simulink model "floating_2_bodies_acc"  (Simulink 6.3)
settings: Solver=ode1  StartTime=0.0  StopTime=inf  FixedStep=0.01  RelTol=1e-6  AbsTol=1e-6
PreLoadFcn:
  | Body_Shv_Double_0661
InitFcn:
  | mech_slider_open_ShV(gcs);
undefined symbols (not defined in the file): Body_01_Inertia, Body_01_Mass, Body_Rt_Inertia, Body_Rt_Mass, deg, Range_of_Ang_degr, s
libraries: mblibv1 x23, simulink x11
settings Model: LastModifiedBy=Alex
settings SimMechanicsCC: VisOnUpdateDiagram=on  VisDuringSimulation=on

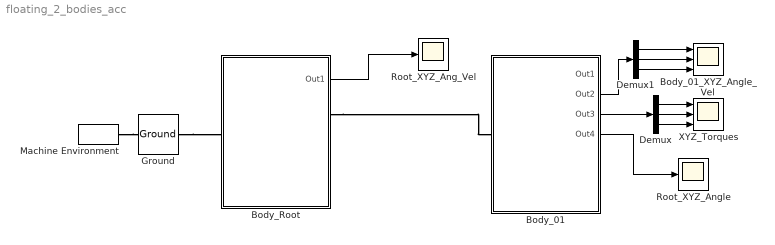
== system floating_2_bodies_acc ==
  Body_01 : Subsystem
  Body_01_XYZ_Angle_Vel : Scope  NumInputPorts=3
      settings: TimeRange=30  YMin=-8e-005~-1~-1  YMax=2e-005~1~1
  Body_Root : Subsystem
  Demux : Demux  Outputs=3
  Demux1 : Demux  Outputs=3
  Ground : mblibv1/Bodies/Ground  LeftPortType=env  RightPortType=workingframe  PhysicalDomain=Mechanical  DialogClass=GroundBlock  CoordPosition=[0 0 0]  CoordPositionUnits=m  StateVectorMgrId=-1  MachineId=[6 1]  ShowEnvPort=on
  Machine Environment : mblibv1/Bodies/Machine Environment  Tag=Factory ground  DialogController=MECH.DialogSource  PortType=env  PhysicalDomain=Mechanical  DialogTemplateClass=MECH.MachineEnvironment  SyncWhenCopied=off  Gravity=[0 0 0]  GravityUnits=m/s^2  GravityAsSignal=off  Dimensionality=Auto-detect  AnalysisType=Forward dynamics  LinearAssemblyTolerance=1e-3  LinearAssemblyToleranceUnits=m  AngularAssemblyTolerance=1e-3  AngularAssemblyToleranceUnits=rad  ConstraintSolverType=Stabilizing  ConstraintRelTolerance=1e-4  ConstraintAbsTolerance=1e-4  UseRobustSingularityHandling=off  StatePerturbationType=Fixed  PerturbationSize=1e-5  VisualizeMachine=on
  Root_XYZ_Ang_Vel : Scope
      settings: TimeRange=60  YMin=-600  YMax=700
  Root_XYZ_Angle : Scope
      settings: TimeRange=10  YMin=-90  YMax=10  SaveName=ScopeData4
  XYZ_Torques : Scope  NumInputPorts=3
      settings: TimeRange=30  YMin=1.01794~-1~-1  YMax=1.01797~1~1  SaveName=ScopeData3
  wires:
  Body_01/3(Out3) -> Demux/1
  Demux/1 -> XYZ_Torques/1
  Demux/2 -> XYZ_Torques/2
  Demux/3 -> XYZ_Torques/3
  Body_01/2(Out2) -> Demux1/1
  Demux1/1 -> Body_01_XYZ_Angle_Vel/1
  Demux1/2 -> Body_01_XYZ_Angle_Vel/2
  Demux1/3 -> Body_01_XYZ_Angle_Vel/3
  Body_Root/1(Out1) -> Root_XYZ_Ang_Vel/1
  Body_01/4(Out4) -> Root_XYZ_Angle/1
  connections:
  Machine Environment/RConn1 -- Ground/LConn1
  Ground/RConn1 -- Body_Root/LConn1
  Body_Root/RConn1 -- Body_01/LConn1

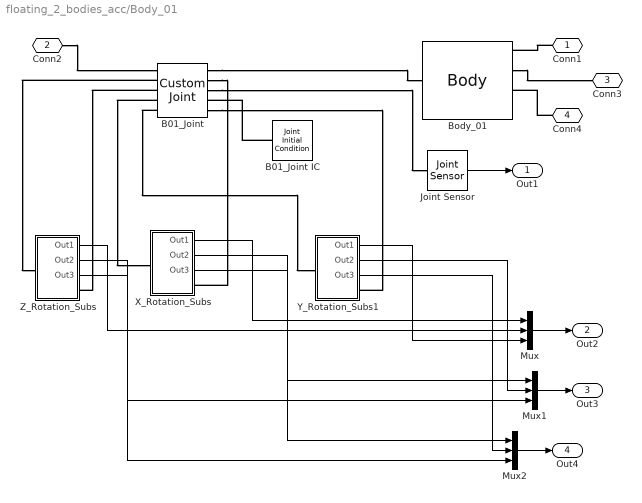
== system floating_2_bodies_acc/Body_01 ==
  B01_Joint : mblibv1/Joints/Custom Joint  PhysicalDomain=mechanical  SubClassName=custom_joint  LeftPortType=blob  RightPortType=blob  LConnTagsString=__newl0|SA1|SA2|SA3|SA4  RConnTagsString=__newr0|SA1|SA2|SA3|SA4  NumSAPorts=8  CutJoint=off  MarkAsCut=off  Primitives=revolute_revolute_revolute  PrimitiveProps=R3$WORLD$[0 0 1]$revolute#R1$WORLD$[1 0 0]$revolute#R2$WORLD$[0 1 0]$revolute  DialogClass=JointBlock
  B01_Joint IC : mblibv1/Sensors &  Actuators/Joint Initial Condition  Orientation=left  PhysicalDomain=mechanical  DialogClass=InitialConditionBlock  InitialConditions=P1$false$0$m$rad$0$m/s$rad/s#P2$false$0$m$rad$0$m/s$rad/s#P3$false$0$m$rad$0$m/s$rad/s#R1$true$X_Ang_Correction$m$deg$Body_01_IVel(1)$m/s$rad/s#R2$true$Body_01_IPos(2)$m$deg$Body_01_IVel(2)$m/s$rad/s#R3$true$Body_01_IPos(3)$m$deg$Body_01_IVel(3)$m/s$rad/s#S$false$0$m$rad$0$m/s$rad/s
  Body_01 : mblibv1/Bodies/Body  PhysicalDomain=mechanical  SubClassName=Unknown  LeftPortType=workingframe  RightPortType=workingframe  LConnTagsString=CS1  RConnTagsString=CS2|CS3|CS4|CS5  DialogClass=MechanicalBodyBlock  Mass=Body_01_Mass  MassUnits=kg  InertiaUnits=kg*m^2  Inertia=Body_01_Inertia  Shape=Cylinder  ShapeDims=[1 1]  ShapeUnits=m  ShapeUse=false  Density=1  DensityUnits=kg/m^3  DensityUse=false  CG=Left$CG$-Body_01_Size$CS1$CS1$m$[0 0 0]$Euler X-Y-Z$deg$ADJOINING$false  WorkingFrames=Left$CS1$[0 0 0]$ADJOINING$ADJOINING$m$[0 0 0]$Euler X-Y-Z$deg$WORLD$true#Right$CS2$-Body_01_Size$CG$CG$m$[0 0 0]$Euler X-Y-Z$deg$WORLD$true#Right$CS3$[-0.5*Body_01_Size(2) -Body_01_Size(2) 0]$CG$CG$m$[0 0 0]$Euler X-Y-Z$deg$WORLD$true#Right$CS4$[0.5*Body_01_Size(2) -Body_01_Size(2) 0]$CG$CG$m$[0 0 0]$Euler X-Y-Z$deg$WORLD$true#Right$CS5$[0 -Body_01_Size(2) -0.2*Body_01_Size(2)]$CG$CG$m$[0 0 0]$Euler X-Y-Z$deg$WORLD$true
  Joint Sensor : mblibv1/Sensors &  Actuators/Joint Sensor  PhysicalDomain=Mechanical  PortType=blob  Muxed=on  Pose=off  Angle=off  AngleUnits=deg  ArcVelocity=on  ArcVelocityUnits=deg/s  ArcAcceleration=off  ArcAccelerationUnits=deg/s^2  CoordPosition=on  CoordPositionUnits=m  Velocity=off  VelocityUnits=m/s  Acceleration=off  AccelerationUnits=m/s^2  Quaternion=on  QuaternionDT=off  QuaternionDDT=off  QuaternionUnits=off  OutputVector=[ 1 ]  ActiveIO=on  Width=1  DialogClass=MechanicalSensorBlock  Primitive=R3  Force=off  ForceUnits=N  Torque=off  TorqueUnits=N-m  ReferenceFrame=Absolute (INERTIAL)  ReactionSensedSide=Base  ReactionReferenceFrame=Local (Body CS)  ReactionForce=off  ReactionForceUnits=N  ReactionMoment=off  ReactionMomentUnits=N-m
  Mux : Mux  Inputs=3
  Mux1 : Mux  Inputs=3
  Mux2 : Mux  Inputs=3
  X_Rotation_Subs : Subsystem
  Y_Rotation_Subs1 : Subsystem
  Z_Rotation_Subs : Subsystem
  Conn1 : PMIOPort  Orientation=left  Port=1  Side=Right
  Conn2 : PMIOPort  Port=2  Side=Left
  Conn3 : PMIOPort  Orientation=left  Port=3  Side=Right
  Conn4 : PMIOPort  Orientation=left  Port=4  Side=Right
  Out1 : Outport
  Out2 : Outport  Port=2
  Out3 : Outport  Port=3
  Out4 : Outport  Port=4
  wires:
  Joint Sensor/1 -> Out1/1
  Z_Rotation_Subs/1(Out1) -> Mux/2
  X_Rotation_Subs/1(Out1) -> Mux/1
  Mux/1 -> Out2/1
  Y_Rotation_Subs1/1(Out1) -> Mux/3
  Mux1/1 -> Out3/1
  X_Rotation_Subs/2(Out2) -> Mux1/1
  Y_Rotation_Subs1/2(Out2) -> Mux1/2
  Z_Rotation_Subs/2(Out2) -> Mux1/3
  Mux2/1 -> Out4/1
  X_Rotation_Subs/3(Out3) -> Mux2/1
  Y_Rotation_Subs1/3(Out3) -> Mux2/2
  Z_Rotation_Subs/3(Out3) -> Mux2/3
  connections:
  B01_Joint/RConn1 -- Body_01/LConn1
  B01_Joint/RConn3 -- Joint Sensor/LConn1
  Conn1/RConn1 -- Body_01/RConn1
  Conn2/RConn1 -- B01_Joint/LConn1
  Conn4/RConn1 -- Body_01/RConn3
  B01_Joint/LConn2 -- Z_Rotation_Subs/LConn1
  B01_Joint/LConn3 -- Z_Rotation_Subs/RConn1
  B01_Joint/LConn4 -- X_Rotation_Subs/LConn1
  B01_Joint/RConn2 -- X_Rotation_Subs/RConn1
  B01_Joint IC/RConn1 -- B01_Joint/RConn4
  B01_Joint/LConn5 -- Y_Rotation_Subs1/LConn1
  B01_Joint/RConn5 -- Y_Rotation_Subs1/RConn1
  Body_01/RConn2 -- Conn3/RConn1

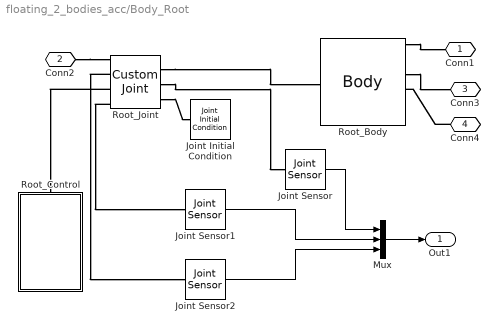
== system floating_2_bodies_acc/Body_Root ==
  Joint Initial Condition : mblibv1/Sensors &  Actuators/Joint Initial Condition  Orientation=left  PhysicalDomain=mechanical  DialogClass=InitialConditionBlock  InitialConditions=P1$true$0$m$rad$Body_Rt_IVel(1)$m/s$rad/s#P2$true$0$m$rad$Body_Rt_IVel(2)$m/s$rad/s#P3$true$0$m$rad$Body_Rt_IVel(3)$m/s$rad/s#R1$true$Body_Rt_IPos(4)$m$deg$Body_Rt_IVel(4)$m/s$rad/s#R2$true$Body_Rt_IPos(5)$m$deg$Body_Rt_IVel(5)$m/s$rad/s#R3$true$Body_Rt_IPos(6)$m$deg$Body_Rt_IVel(6)$m/s$rad/s#S$false$0$m$rad$0$m/s$rad/s
  Joint Sensor : mblibv1/Sensors &  Actuators/Joint Sensor  PhysicalDomain=Mechanical  PortType=blob  Muxed=on  Pose=off  Angle=off  AngleUnits=deg  ArcVelocity=on  ArcVelocityUnits=deg/s  ArcAcceleration=off  ArcAccelerationUnits=deg/s^2  CoordPosition=on  CoordPositionUnits=m  Velocity=off  VelocityUnits=m/s  Acceleration=off  AccelerationUnits=m/s^2  Quaternion=on  QuaternionDT=off  QuaternionDDT=off  QuaternionUnits=off  OutputVector=[ 1 ]  ActiveIO=on  Width=1  DialogClass=MechanicalSensorBlock  Primitive=R1  Force=off  ForceUnits=N  Torque=off  TorqueUnits=N-m  ReferenceFrame=Absolute (INERTIAL)  ReactionSensedSide=Base  ReactionReferenceFrame=Local (Body CS)  ReactionForce=off  ReactionForceUnits=N  ReactionMoment=off  ReactionMomentUnits=N-m
  Joint Sensor1 : mblibv1/Sensors &  Actuators/Joint Sensor  PhysicalDomain=Mechanical  PortType=blob  Muxed=on  Pose=off  Angle=off  AngleUnits=deg  ArcVelocity=on  ArcVelocityUnits=deg/s  ArcAcceleration=off  ArcAccelerationUnits=deg/s^2  CoordPosition=on  CoordPositionUnits=m  Velocity=off  VelocityUnits=m/s  Acceleration=off  AccelerationUnits=m/s^2  Quaternion=on  QuaternionDT=off  QuaternionDDT=off  QuaternionUnits=off  OutputVector=[ 1 ]  ActiveIO=on  Width=1  DialogClass=MechanicalSensorBlock  Primitive=R2  Force=off  ForceUnits=N  Torque=off  TorqueUnits=N-m  ReferenceFrame=Absolute (INERTIAL)  ReactionSensedSide=Base  ReactionReferenceFrame=Local (Body CS)  ReactionForce=off  ReactionForceUnits=N  ReactionMoment=off  ReactionMomentUnits=N-m
  Joint Sensor2 : mblibv1/Sensors &  Actuators/Joint Sensor  PhysicalDomain=Mechanical  PortType=blob  Muxed=on  Pose=off  Angle=off  AngleUnits=deg  ArcVelocity=on  ArcVelocityUnits=deg/s  ArcAcceleration=off  ArcAccelerationUnits=deg/s^2  CoordPosition=on  CoordPositionUnits=m  Velocity=off  VelocityUnits=m/s  Acceleration=off  AccelerationUnits=m/s^2  Quaternion=on  QuaternionDT=off  QuaternionDDT=off  QuaternionUnits=off  OutputVector=[ 1 ]  ActiveIO=on  Width=1  DialogClass=MechanicalSensorBlock  Primitive=R3  Force=off  ForceUnits=N  Torque=off  TorqueUnits=N-m  ReferenceFrame=Absolute (INERTIAL)  ReactionSensedSide=Base  ReactionReferenceFrame=Local (Body CS)  ReactionForce=off  ReactionForceUnits=N  ReactionMoment=off  ReactionMomentUnits=N-m
  Mux : Mux  Inputs=3
  Root_Body : mblibv1/Bodies/Body  PhysicalDomain=mechanical  SubClassName=Unknown  LeftPortType=workingframe  RightPortType=workingframe  LConnTagsString=CG  RConnTagsString=CS1|CS2|CS3|CS4|CS5|CS6  DialogClass=MechanicalBodyBlock  Mass=Body_Rt_Mass  MassUnits=kg  InertiaUnits=kg*m^2  Inertia=Body_Rt_Inertia  Shape=Cylinder  ShapeDims=[1 1]  ShapeUnits=m  ShapeUse=false  Density=1  DensityUnits=kg/m^3  DensityUse=false  CG=Left$CG$Body_Rt_IPos(1:3)$WORLD$WORLD$m$[0 0 0]$Euler X-Y-Z$deg$WORLD$true  WorkingFrames=Right$CS1$Body_Rt_Size$CG$CG$m$[0 0 0]$Euler X-Y-Z$deg$WORLD$true#Right$CS2$[0 -Body_Rt_Size(2) 0]$CG$CG$m$[0 0 0]$Euler X-Y-Z$deg$WORLD$true#Right$CS3$[-0.4*Body_Rt_Size(2) Body_Rt_Size(2) 0]$CG$CG$m$[0 0 0]$Euler X-Y-Z$deg$WORLD$true#Right$CS4$[0.4*Body_Rt_Size(2) Body_Rt_Size(2) 0]$CG$CG$m$[0 0 0]$Euler X-Y-Z$deg$WORLD$true#Right$CS5$[0 Body_Rt_Size(2) -0.2*Body_Rt_Size(2)]$CG$CG$m$[0 0 0]$Euler X-Y-Z$deg$WORLD$true#Right$CS6$-CM_loc_Rel_Rt$CG$CG$m$[0 0 0]$Euler X-Y-Z$deg$WORLD$true
  Root_Control : Subsystem  Orientation=down
  Root_Joint : mblibv1/Joints/Custom Joint  PhysicalDomain=mechanical  SubClassName=custom_joint  LeftPortType=blob  RightPortType=blob  LConnTagsString=__newl0|SA1|SA2|SA3  RConnTagsString=__newr0|SA1|SA2  NumSAPorts=5  CutJoint=off  MarkAsCut=off  Primitives=prismatic_prismatic_prismatic_revolute_revolute_revolute  PrimitiveProps=P1$WORLD$[1 0 0]$prismatic#P2$WORLD$[0 1 0]$prismatic#P3$WORLD$[0 0 1]$prismatic#R1$WORLD$[1 0 0]$revolute#R2$WORLD$[0 1 0]$revolute#R3$WORLD$[0 0 1]$revolute  DialogClass=JointBlock
  Conn1 : PMIOPort  Orientation=left  Port=1  Side=Right
  Conn2 : PMIOPort  Port=2  Side=Left
  Conn3 : PMIOPort  Orientation=left  Port=3  Side=Right
  Conn4 : PMIOPort  Orientation=left  Port=4  Side=Right
  Out1 : Outport
  wires:
  Mux/1 -> Out1/1
  Joint Sensor/1 -> Mux/1
  Joint Sensor1/1 -> Mux/2
  Joint Sensor2/1 -> Mux/3
  connections:
  Root_Joint/RConn2 -- Joint Sensor/LConn1
  Conn2/RConn1 -- Root_Joint/LConn1
  Conn4/RConn1 -- Root_Body/RConn4
  Root_Body/RConn3 -- Conn3/RConn1
  Root_Joint/RConn1 -- Root_Body/LConn1
  Root_Body/RConn1 -- Conn1/RConn1
  Root_Joint/RConn3 -- Joint Initial Condition/RConn1
  Root_Joint/LConn3 -- Root_Control/LConn1
  Root_Joint/LConn2 -- Joint Sensor2/LConn1
  Root_Joint/LConn4 -- Joint Sensor1/LConn1

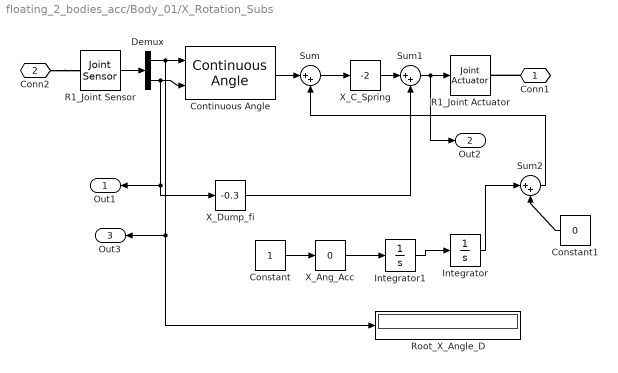
== system floating_2_bodies_acc/Body_01/X_Rotation_Subs ==
  Constant : Constant
  Constant1 : Constant  Orientation=left  Value=0
  Continuous Angle : mblibv1/Utilities/Continuous Angle  Tag=Factory continuousAngle  rad=deg  rads=deg/s
  Demux : Demux  Outputs=2
  Integrator : Integrator  LimitOutput=on  UpperSaturationLimit=Range_of_Ang_degr(2,1)  LowerSaturationLimit=Range_of_Ang_degr(1,1)
  Integrator1 : Integrator  LimitOutput=on  UpperSaturationLimit=200  LowerSaturationLimit=-200
  R1_Joint Actuator : mblibv1/Sensors &  Actuators/Joint Actuator  PhysicalDomain=Mechanical  PortType=blob  ActuationStyle=Force  AngleUnits=deg  ArcVelocityUnits=deg/s  ArcAccelerationUnits=deg/s^2  CoordPositionUnits=m  VelocityUnits=m/s  AccelerationUnits=m/s^2  ForceUnits=N  TorqueUnits=N-m  ActiveIO=on  Width=1  DialogClass=MechanicalActuatorBlock  Primitive=R1  ReferenceFrame=Absolute (INERTIAL)
  R1_Joint Sensor : mblibv1/Sensors &  Actuators/Joint Sensor  PhysicalDomain=Mechanical  PortType=blob  Muxed=on  Pose=off  Angle=on  AngleUnits=deg  ArcVelocity=on  ArcVelocityUnits=deg/s  ArcAcceleration=off  ArcAccelerationUnits=deg/s^2  CoordPosition=on  CoordPositionUnits=m  Velocity=off  VelocityUnits=m/s  Acceleration=off  AccelerationUnits=m/s^2  Quaternion=on  QuaternionDT=off  QuaternionDDT=off  QuaternionUnits=off  OutputVector=[ 1 1 ]  ActiveIO=on  Width=2  DialogClass=MechanicalSensorBlock  Primitive=R1  Force=off  ForceUnits=N  Torque=off  TorqueUnits=N-m  ReferenceFrame=Absolute (INERTIAL)  ReactionSensedSide=Base  ReactionReferenceFrame=Local (Body CS)  ReactionForce=off  ReactionForceUnits=N  ReactionMoment=off  ReactionMomentUnits=N-m
  Root_X_Angle_D : Display
  Sum : Sum  Inputs=|++
  Sum1 : Sum  Inputs=|++
  Sum2 : Sum  Inputs=|++
  X_Ang_Acc : simulink/Math Operations/Slider Gain  Tag=Start_Open  low=-1000  gain=0  high=1000
  X_C_Spring : simulink/Math Operations/Slider Gain  low=-2  gain=-2  high=0
  X_Dump_fi : simulink/Math Operations/Slider Gain  low=-0.3  gain=-0.3  high=0
  Conn1 : PMIOPort  Orientation=left  Port=1  Side=Right
  Conn2 : PMIOPort  Port=2  Side=Left
  Out1 : Outport  Orientation=left
  Out2 : Outport  Port=2
  Out3 : Outport  Orientation=left  Port=3
  wires:
  R1_Joint Sensor/1 -> Demux/1
  X_Dump_fi/1 -> Sum1/2
  Constant/1 -> X_Ang_Acc/1
  Sum/1 -> X_C_Spring/1
  X_C_Spring/1 -> Sum1/1
  Demux/1 -> Continuous Angle/1, Root_X_Angle_D/1, Out3/1
  Continuous Angle/1 -> Sum/1
  Demux/2 -> Continuous Angle/2, X_Dump_fi/1, Out1/1
  Sum1/1 -> R1_Joint Actuator/1, Out2/1
  Constant1/1 -> Sum2/2
  Integrator/1 -> Sum2/1
  Sum2/1 -> Sum/2
  Integrator1/1 -> Integrator/1
  X_Ang_Acc/1 -> Integrator1/1
  connections:
  Conn1/RConn1 -- R1_Joint Actuator/RConn1
  Conn2/RConn1 -- R1_Joint Sensor/LConn1

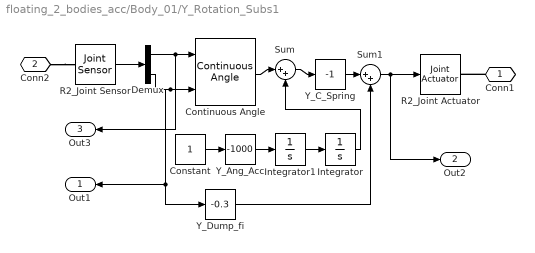
== system floating_2_bodies_acc/Body_01/Y_Rotation_Subs1 ==
  Constant : Constant
  Continuous Angle : mblibv1/Utilities/Continuous Angle  Tag=Factory continuousAngle  rad=deg  rads=deg/s
  Demux : Demux  Outputs=2
  Integrator : Integrator  LimitOutput=on  UpperSaturationLimit=Range_of_Ang_degr(2,2)  LowerSaturationLimit=Range_of_Ang_degr(1,2)
  Integrator1 : Integrator  LimitOutput=on  UpperSaturationLimit=200  LowerSaturationLimit=-200
  R2_Joint Actuator : mblibv1/Sensors &  Actuators/Joint Actuator  PhysicalDomain=Mechanical  PortType=blob  ActuationStyle=Force  AngleUnits=deg  ArcVelocityUnits=deg/s  ArcAccelerationUnits=deg/s^2  CoordPositionUnits=m  VelocityUnits=m/s  AccelerationUnits=m/s^2  ForceUnits=N  TorqueUnits=N-m  ActiveIO=on  Width=1  DialogClass=MechanicalActuatorBlock  Primitive=R2  ReferenceFrame=Absolute (INERTIAL)
  R2_Joint Sensor : mblibv1/Sensors &  Actuators/Joint Sensor  PhysicalDomain=Mechanical  PortType=blob  Muxed=on  Pose=off  Angle=on  AngleUnits=deg  ArcVelocity=on  ArcVelocityUnits=deg/s  ArcAcceleration=off  ArcAccelerationUnits=deg/s^2  CoordPosition=on  CoordPositionUnits=m  Velocity=off  VelocityUnits=m/s  Acceleration=off  AccelerationUnits=m/s^2  Quaternion=on  QuaternionDT=off  QuaternionDDT=off  QuaternionUnits=off  OutputVector=[ 1 1 ]  ActiveIO=on  Width=2  DialogClass=MechanicalSensorBlock  Primitive=R2  Force=off  ForceUnits=N  Torque=off  TorqueUnits=N-m  ReferenceFrame=Absolute (INERTIAL)  ReactionSensedSide=Base  ReactionReferenceFrame=Local (Body CS)  ReactionForce=off  ReactionForceUnits=N  ReactionMoment=off  ReactionMomentUnits=N-m
  Sum : Sum  Inputs=|++
  Sum1 : Sum  Inputs=|++
  Y_Ang_Acc : simulink/Math Operations/Slider Gain  Tag=Start_Open  low=-1000  gain=-1000  high=1000
  Y_C_Spring : simulink/Math Operations/Slider Gain  low=-1  gain=-1  high=0
  Y_Dump_fi : simulink/Math Operations/Slider Gain  low=-0.3  gain=-0.3  high=0
  Conn1 : PMIOPort  Orientation=left  Port=1  Side=Right
  Conn2 : PMIOPort  Port=2  Side=Left
  Out1 : Outport  Orientation=left
  Out2 : Outport  Port=2
  Out3 : Outport  Orientation=left  Port=3
  wires:
  R2_Joint Sensor/1 -> Demux/1
  Demux/2 -> Continuous Angle/2, Y_Dump_fi/1, Out1/1
  Y_Dump_fi/1 -> Sum1/2
  Sum1/1 -> R2_Joint Actuator/1, Out2/1
  Constant/1 -> Y_Ang_Acc/1
  Sum/1 -> Y_C_Spring/1
  Y_C_Spring/1 -> Sum1/1
  Demux/1 -> Continuous Angle/1, Out3/1
  Continuous Angle/1 -> Sum/1
  Integrator/1 -> Sum/2
  Y_Ang_Acc/1 -> Integrator1/1
  Integrator1/1 -> Integrator/1
  connections:
  Conn1/RConn1 -- R2_Joint Actuator/RConn1
  Conn2/RConn1 -- R2_Joint Sensor/LConn1

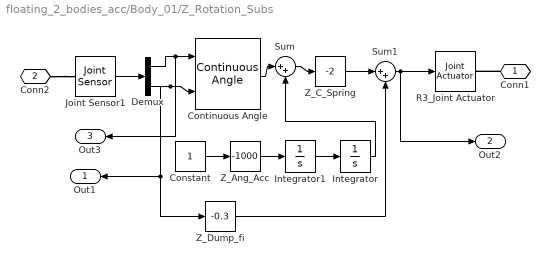
== system floating_2_bodies_acc/Body_01/Z_Rotation_Subs ==
  Constant : Constant
  Continuous Angle : mblibv1/Utilities/Continuous Angle  Tag=Factory continuousAngle  rad=deg  rads=deg/s
  Demux : Demux  Outputs=2
  Integrator : Integrator  LimitOutput=on  UpperSaturationLimit=Range_of_Ang_degr(2,3)  LowerSaturationLimit=Range_of_Ang_degr(1,3)
  Integrator1 : Integrator  LimitOutput=on  UpperSaturationLimit=200  LowerSaturationLimit=-200
  Joint Sensor1 : mblibv1/Sensors &  Actuators/Joint Sensor  PhysicalDomain=Mechanical  PortType=blob  Muxed=on  Pose=off  Angle=on  AngleUnits=deg  ArcVelocity=on  ArcVelocityUnits=deg/s  ArcAcceleration=off  ArcAccelerationUnits=deg/s^2  CoordPosition=on  CoordPositionUnits=m  Velocity=off  VelocityUnits=m/s  Acceleration=off  AccelerationUnits=m/s^2  Quaternion=on  QuaternionDT=off  QuaternionDDT=off  QuaternionUnits=off  OutputVector=[ 1 1 ]  ActiveIO=on  Width=2  DialogClass=MechanicalSensorBlock  Primitive=R3  Force=off  ForceUnits=N  Torque=off  TorqueUnits=N-m  ReferenceFrame=Absolute (INERTIAL)  ReactionSensedSide=Base  ReactionReferenceFrame=Local (Body CS)  ReactionForce=off  ReactionForceUnits=N  ReactionMoment=off  ReactionMomentUnits=N-m
  R3_Joint Actuator : mblibv1/Sensors &  Actuators/Joint Actuator  PhysicalDomain=Mechanical  PortType=blob  ActuationStyle=Force  AngleUnits=deg  ArcVelocityUnits=deg/s  ArcAccelerationUnits=deg/s^2  CoordPositionUnits=m  VelocityUnits=m/s  AccelerationUnits=m/s^2  ForceUnits=N  TorqueUnits=N-m  ActiveIO=on  Width=1  DialogClass=MechanicalActuatorBlock  Primitive=R3  ReferenceFrame=Absolute (INERTIAL)
  Sum : Sum  Inputs=|++
  Sum1 : Sum  Inputs=|++
  "Z_Ang_Acc " : simulink/Math Operations/Slider Gain  Tag=Start_Open  low=-1000  gain=-1000  high=1000
  "Z_C_Spring " : simulink/Math Operations/Slider Gain  low=-2  gain=-2  high=0
  Z_Dump_fi : simulink/Math Operations/Slider Gain  low=-0.3  gain=-0.3  high=0
  Conn1 : PMIOPort  Orientation=left  Port=1  Side=Right
  Conn2 : PMIOPort  Port=2  Side=Left
  Out1 : Outport  Orientation=left
  Out2 : Outport  Port=2
  Out3 : Outport  Orientation=left  Port=3
  wires:
  Joint Sensor1/1 -> Demux/1
  Demux/2 -> Continuous Angle/2, Z_Dump_fi/1, Out1/1
  Z_Dump_fi/1 -> Sum1/2
  Sum1/1 -> R3_Joint Actuator/1, Out2/1
  Constant/1 -> "Z_Ang_Acc "/1
  Sum/1 -> "Z_C_Spring "/1
  "Z_C_Spring "/1 -> Sum1/1
  Demux/1 -> Continuous Angle/1, Out3/1
  Continuous Angle/1 -> Sum/1
  Integrator/1 -> Sum/2
  "Z_Ang_Acc "/1 -> Integrator1/1
  Integrator1/1 -> Integrator/1
  connections:
  Conn1/RConn1 -- R3_Joint Actuator/RConn1
  Conn2/RConn1 -- Joint Sensor1/LConn1

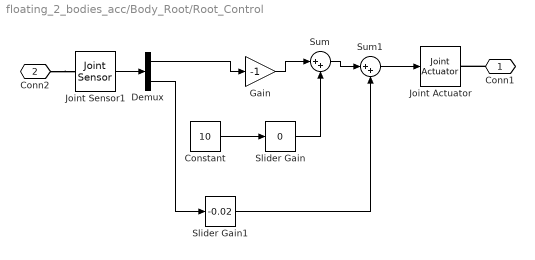
== system floating_2_bodies_acc/Body_Root/Root_Control ==
  Constant : Constant  Value=10
  Demux : Demux  Outputs=2
  Gain : Gain  Gain=-1
  Joint Actuator : mblibv1/Sensors &  Actuators/Joint Actuator  PhysicalDomain=Mechanical  PortType=blob  ActuationStyle=Force  AngleUnits=deg  ArcVelocityUnits=deg/s  ArcAccelerationUnits=deg/s^2  CoordPositionUnits=m  VelocityUnits=m/s  AccelerationUnits=m/s^2  ForceUnits=N  TorqueUnits=N-m  ActiveIO=off  Width=1  DialogClass=MechanicalActuatorBlock  Primitive=R1  ReferenceFrame=Absolute (INERTIAL)
  Joint Sensor1 : mblibv1/Sensors &  Actuators/Joint Sensor  PhysicalDomain=Mechanical  PortType=blob  Muxed=on  Pose=off  Angle=on  AngleUnits=deg  ArcVelocity=on  ArcVelocityUnits=deg/s  ArcAcceleration=off  ArcAccelerationUnits=deg/s^2  CoordPosition=on  CoordPositionUnits=m  Velocity=off  VelocityUnits=m/s  Acceleration=off  AccelerationUnits=m/s^2  Quaternion=on  QuaternionDT=off  QuaternionDDT=off  QuaternionUnits=off  OutputVector=[ 1 1 ]  ActiveIO=on  Width=2  DialogClass=MechanicalSensorBlock  Primitive=R3  Force=off  ForceUnits=N  Torque=off  TorqueUnits=N-m  ReferenceFrame=Absolute (INERTIAL)  ReactionSensedSide=Base  ReactionReferenceFrame=Local (Body CS)  ReactionForce=off  ReactionForceUnits=N  ReactionMoment=off  ReactionMomentUnits=N-m
  Slider Gain : simulink/Math Operations/Slider Gain  low=0  gain=0  high=15
  Slider Gain1 : simulink/Math Operations/Slider Gain  low=-0.02  gain=-0.02  high=0
  Sum : Sum  Inputs=|++
  Sum1 : Sum  Inputs=|++
  Conn1 : PMIOPort  Orientation=left  Port=1  Side=Right
  Conn2 : PMIOPort  Port=2  Side=Left
  wires:
  Gain/1 -> Sum/1
  Joint Sensor1/1 -> Demux/1
  Demux/1 -> Gain/1
  Sum/1 -> Sum1/1
  Demux/2 -> Slider Gain1/1
  Slider Gain1/1 -> Sum1/2
  Sum1/1 -> Joint Actuator/1
  Constant/1 -> Slider Gain/1
  Slider Gain/1 -> Sum/2
  connections:
  Conn1/RConn1 -- Joint Actuator/RConn1
  Conn2/RConn1 -- Joint Sensor1/LConn1
